simulink model "test_motors"  (R2023a)
settings: Solver=FixedStepAuto  StartTime=0.0  StopTime=inf  FixedStep=0.01  RelTol=1e-3  EnableMultiTasking=on
undefined symbols (not defined in the file): AUX, dev, Main, pwm_output0, pwm_output1
libraries: px4Sensorslib x10, px4lib x2, px4uORBlib x1, simulink x1
settings Model: SimulationMode=external  ExtModeTrigDuration=10  Creator=ArriGE66  LastModifiedBy=User
settings SolverCC: PositivePriorityOrder=on
settings OptimizationCC: EnhancedBackFolding=on  PassReuseOutputArgsAs=Individual arguments  ZeroExternalMemoryAtStartup=off  ZeroInternalMemoryAtStartup=off  MaxStackSize=64  OptimizeBlockOrder=speed  DifferentSizesBufferReuse=on  OptimizationCustomize=off  EfficientTunableParamExpr=on
settings DebuggingCC: ParameterTunabilityLossMsg=error
settings HardwareCC: ProdBitPerPointer=32  ProdBitPerSizeT=32  ProdBitPerPtrDiffT=32  ProdLargestAtomicInteger=Long  ProdLargestAtomicFloat=Double  ProdWordSize=32  ProdLongLongMode=on  ProdHWDeviceType=ARM Compatible->ARM Cortex
settings SFSimCC: MATLABDynamicMemAlloc=off  SimTargetLang=C++
settings RTWCC: Description=Embedded Coder  SystemTargetFile=ert.tlc  HardwareBoard=PX4 Cube Orange  TemplateMakefile=ert_default_tmf  Toolchain=GNU Tools for PX4 Autopilots  TargetLang=C++
settings CodeAppCC: ForceParamTrailComments=on  IgnoreCustomStorageClasses=off  OperatorAnnotations=on  SimulinkDataObjDesc=on  SFDataObjDesc=on  InsertBlockDesc=on
settings ERTTargetCC: ExtMode=on  ExtModeTransport=3  ExtModeStaticAlloc=on  ExtModeStaticAllocSize=1024  ExtModeMexFile=ext_xcp  ExtModeMexArgs=1 COM10 3000000  ExtModeIntrfLevel=Level2 - Open

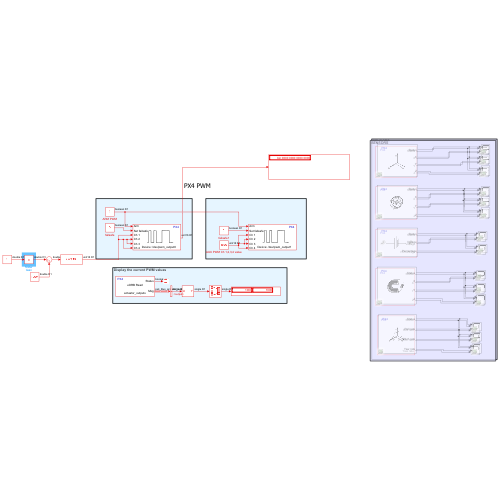
[thumbnail: Simulink's stored preview of the top-level diagram]
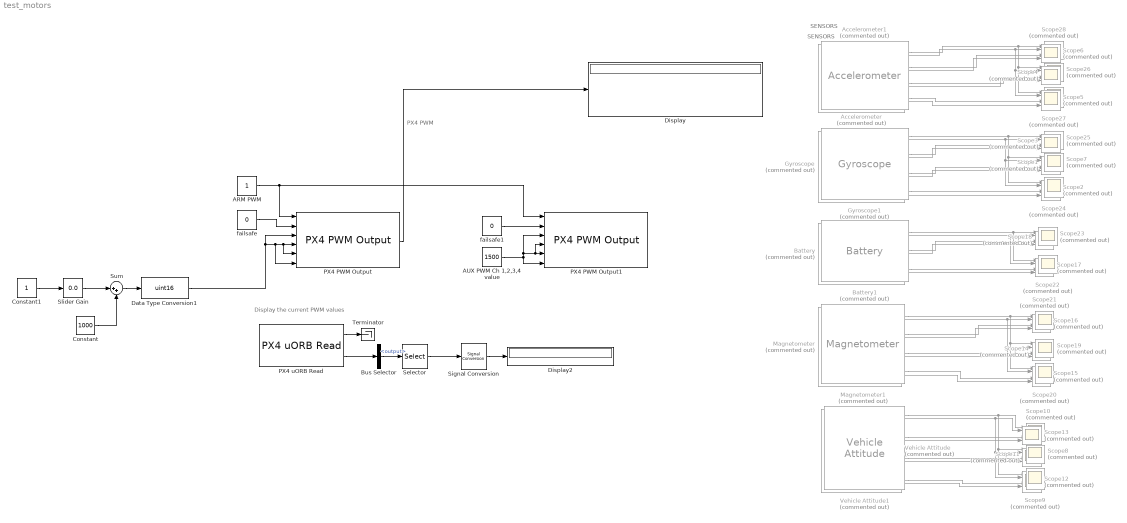
== system test_motors ==
  note: PX4 PWM
  note: Display the current PWM values
  note: SENSORS
  note: SENSORS
  ARM PWM : Constant  OutDataTypeStr=boolean  SampleTime=0.01
  AUX PWM Ch 1,2,3,4 value : Constant  Value=1500  OutDataTypeStr=uint16  SampleTime=0.01
  Accelerometer : px4Sensorslib/Accelerometer  Commented=on  uorbTimeStamp=off  BlockingMode=off  BlockTimeout=1e-3  sampleTime=1/100
  Accelerometer1 : px4Sensorslib/Accelerometer  Commented=on  uorbTimeStamp=off  BlockingMode=off  BlockTimeout=1e-3  sampleTime=1/100
  Battery : px4Sensorslib/Battery  Commented=on  voltage=on  current=off  remaining=on  warning=off  timestamp=off  sampleTime=1/100  BlockingMode=off  BlockTimeout=1e-3
  Battery1 : px4Sensorslib/Battery  Commented=on  voltage=on  current=off  remaining=on  warning=off  timestamp=off  sampleTime=1/100  BlockingMode=off  BlockTimeout=1e-3
  Bus Selector : BusSelector  OutputSignals=output
  Constant : Constant  Value=1000  SampleTime=0.01
  Constant1 : Constant  SampleTime=0.01
  Data Type Conversion1 : DataTypeConversion  OutDataTypeStr=uint16  SaturateOnIntegerOverflow=off  RndMeth=Floor
  Display : Display
      settings: Format=binary (Stored Integer)
  Display2 : Display
  Gyroscope : px4Sensorslib/Gyroscope  Commented=on  uorbTimeStamp=off  BlockingMode=off  BlockTimeout=1e-3  sampleTime=1/100
  Gyroscope1 : px4Sensorslib/Gyroscope  Commented=on  uorbTimeStamp=off  BlockingMode=off  BlockTimeout=1e-3  sampleTime=1/100
  Magnetometer : px4Sensorslib/Magnetometer  Commented=on  uorbTimeStamp=off  BlockingMode=off  BlockTimeout=1e-3  sampleTime=1/100
  Magnetometer1 : px4Sensorslib/Magnetometer  Commented=on  uorbTimeStamp=off  BlockingMode=off  BlockTimeout=1e-3  sampleTime=1/100
  PX4 PWM Output : px4lib/PX4 PWM Output  pwmDevice=Main (/dev/pwm_output0)  pwmChannel1_=on  pwmChannel2_=on  pwmChannel3_=on  pwmChannel4_=on  pwmChannel5_=off  pwmChannel6_=off  pwmChannel7_=off  pwmChannel8_=off  forceTerminateFailsafe=off  outputErrorStatus=on
  PX4 PWM Output1 : px4lib/PX4 PWM Output  pwmDevice=AUX (/dev/pwm_output1)  pwmChannel1_=on  pwmChannel2_=on  pwmChannel3_=on  pwmChannel4_=on  pwmChannel5_=off  pwmChannel6_=off  pwmChannel7_=off  pwmChannel8_=off  forceTerminateFailsafe=off  outputErrorStatus=off
  PX4 uORB Read : px4uORBlib/PX4 uORB Read  uORBTopic=actuator_outputs  selectInstance=actuator_outputs  SampleTime=0.01  BlockingMode=off  BlockTimeout=1e-3
  Scope{1..28} (28 alike) : Scope  Commented=on  NumInputPorts=2
  Selector : Selector  InputPortWidth=16  IndexOptions=Index vector (dialog)  Indices=[1 2]  OutputSizes=1
  Signal Conversion : SignalConversion  OverrideOpt=off
  Slider Gain : simulink/Math Operations/Slider Gain  gain=0.0  low=0  high=1000
  Sum : Sum  Inputs=|++
  Terminator : Terminator
  Vehicle Attitude : px4Sensorslib/Vehicle Attitude  Commented=on  rollRate=on  pitchRate=on  yawRate=on  quaternion=off  uorbTimeStamp=off  BlockingMode=off  BlockTimeout=0.001  sampleTime=1/100
  Vehicle Attitude1 : px4Sensorslib/Vehicle Attitude  Commented=on  rollRate=on  pitchRate=on  yawRate=on  quaternion=off  uorbTimeStamp=off  BlockingMode=off  BlockTimeout=0.001  sampleTime=1/100
  failsafe : Constant  Value=0  OutDataTypeStr=boolean  SampleTime=0.01
  failsafe1 : Constant  Value=0  OutDataTypeStr=boolean  SampleTime=0.01
  wires:
  ARM PWM/1 -> PX4 PWM Output1/1, PX4 PWM Output/1
  Data Type Conversion1/1 -> PX4 PWM Output/6, PX4 PWM Output/5, PX4 PWM Output/4, PX4 PWM Output/3
  Bus Selector/1 -> Selector/1  "<output>"
  PX4 uORB Read/1 -> Terminator/1
  failsafe/1 -> PX4 PWM Output/2
  Selector/1 -> Signal Conversion/1
  AUX PWM Ch 1,2,3,4 value/1 -> PX4 PWM Output1/3, PX4 PWM Output1/5, PX4 PWM Output1/4, PX4 PWM Output1/6
  PX4 uORB Read/2 -> Bus Selector/1
  failsafe1/1 -> PX4 PWM Output1/2
  Signal Conversion/1 -> Display2/1
  Slider Gain/1 -> Sum/1
  Constant/1 -> Sum/2
  Constant1/1 -> Slider Gain/1
  Sum/1 -> Data Type Conversion1/1
  PX4 PWM Output/1 -> Display/1
  Accelerometer/4 -> Scope5/2
  Gyroscope/2 -> Scope3/2
  Battery/3 -> Scope17/2
  Accelerometer/1 -> Scope5/1, Scope4/1, Scope6/1
  Vehicle Attitude/2 -> Scope13/2
  Vehicle Attitude/3 -> Scope11/2
  Vehicle Attitude/4 -> Scope12/2
  Magnetometer/3 -> Scope14/2
  Gyroscope/1 -> Scope2/1, Scope1/1, Scope3/1
  Battery/2 -> Scope18/2
  Gyroscope/3 -> Scope1/2
  Magnetometer/4 -> Scope15/2
  Vehicle Attitude/1 -> Scope12/1, Scope11/1, Scope13/1
  Accelerometer/2 -> Scope6/2
  Magnetometer/1 -> Scope15/1, Scope14/1, Scope16/1
  Gyroscope/4 -> Scope2/2
  Magnetometer/2 -> Scope16/2
  Accelerometer/3 -> Scope4/2
  Battery/1 -> Scope17/1, Scope18/1
  Battery1/1 -> Scope23/1, Scope22/1
  Accelerometer1/3 -> Scope26/2
  Magnetometer1/2 -> Scope21/2
  Gyroscope1/4 -> Scope24/2
  Magnetometer1/1 -> Scope21/1, Scope19/1, Scope20/1
  Accelerometer1/2 -> Scope28/2
  Vehicle Attitude1/1 -> Scope10/1, Scope8/1, Scope9/1
  Magnetometer1/4 -> Scope20/2
  Gyroscope1/3 -> Scope7/2
  Battery1/2 -> Scope23/2
  Gyroscope1/1 -> Scope25/1, Scope7/1, Scope24/1
  Magnetometer1/3 -> Scope19/2
  Vehicle Attitude1/4 -> Scope9/2
  Vehicle Attitude1/3 -> Scope8/2
  Vehicle Attitude1/2 -> Scope10/2
  Accelerometer1/1 -> Scope28/1, Scope26/1, Scope27/1
  Battery1/3 -> Scope22/2
  Gyroscope1/2 -> Scope25/2
  Accelerometer1/4 -> Scope27/2
